simulink model "Ex7_4"  (Simulink 6.0)
settings: Solver=ode4  SolverMode=SingleTasking  StartTime=0.0  StopTime=200*Ts  RelTol=1e-3  AbsTol=1e-6
undefined symbols (not defined in the file or in its folder): Ampl, finrad, gainerror, offset, phasejitter, Ts
libraries: simulink x2
settings Model: Creator=francomaloberti  LastModifiedBy=Cri  ExtModeAutoUpdateStatusClock=off
settings DataIOCC: LimitDataPoints=off  SignalLoggingName=sigsOut
settings OptimizationCC: BooleanDataType=off  InlineInvariantSignals=off
settings DebuggingCC: SolverPrmCheckMsg=none
settings HardwareCC: TargetUnknown=on

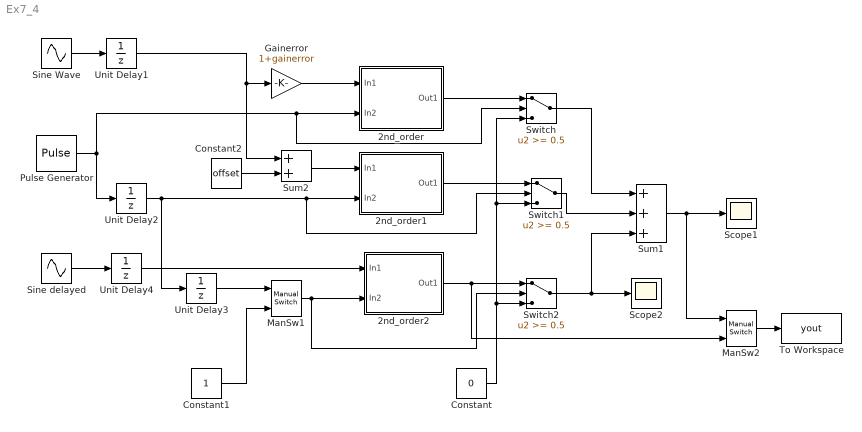
== system Ex7_4 ==
  2nd_order : Subsystem
      mask Display:
      | plot([20 10 20 10 20 30 40 20], [35 35 25 15 15 35 15 15])
      | port_label('input', 1, 'in');
      | port_label('input', 2, 'ck')
  2nd_order1 : Subsystem
      mask Display:
      | plot([20 10 20 10 20 30 40 20], [35 35 25 15 15 35 15 15])
      | port_label('input', 1, 'in');
      | port_label('input', 2, 'ck')
  2nd_order2 : Subsystem
      mask Display:
      | plot([20 10 20 10 20 30 40 20], [35 35 25 15 15 35 15 15])
      | port_label('input', 1, 'in');
      | port_label('input', 2, 'ck')
  Constant : Constant  Value=0
  Constant1 : Constant
  Constant2 : Constant  Value=offset
  Gainerror : Gain  Gain=1+gainerror
  ManSw1 : simulink/Signal Routing/Manual Switch  sw=1  action=0
  ManSw2 : simulink/Signal Routing/Manual Switch  sw=1  action=0
  Pulse Generator : DiscretePulseGenerator  PulseType=Time based  Period=3*Ts  PulseWidth=100/3
  Scope1 : Scope
      settings: TickLabels=on  DataFormat=Array
  Scope2 : Scope
      settings: TickLabels=on  SaveName=ScopeData2  DataFormat=Array
  Sine Wave : Sin  Amplitude=Ampl  Frequency=finrad  SampleTime=0
  Sine delayed : Sin  Amplitude=Ampl  Frequency=finrad  Phase=phasejitter  SampleTime=0
  Sum1 : Sum  Inputs=+++  SaturateOnIntegerOverflow=on  InputSameDT=on
  Sum2 : Sum  SaturateOnIntegerOverflow=on  InputSameDT=on
  Switch : Switch  Threshold=0.5
  Switch1 : Switch  Threshold=0.5
  Switch2 : Switch  Threshold=0.5
  To Workspace : ToWorkspace  VariableName=yout  SampleTime=-1  SaveFormat=Array
  Unit Delay{1..4} (4 alike) : UnitDelay  SampleTime=Ts
  wires:
  Sine Wave/1 -> Unit Delay1/1
  Pulse Generator/1 -> Unit Delay2/1, 2nd_order/2(In2), Switch/2
  Unit Delay1/1 -> Sum2/1, Gainerror/1
  Sum1/1 -> Scope1/1, ManSw2/1
  2nd_order/1(Out1) -> Switch/1
  2nd_order1/1(Out1) -> Switch1/1
  2nd_order2/1(Out1) -> ManSw2/2, Switch2/1
  Switch/1 -> Sum1/1
  Switch1/1 -> Sum1/2
  Constant/1 -> Switch2/3, Switch1/3, Switch/3
  Switch2/1 -> Scope2/1, Sum1/3
  Unit Delay2/1 -> Unit Delay3/1, Switch1/2, 2nd_order1/2(In2)
  ManSw1/1 -> Switch2/2, 2nd_order2/2(In2)
  Unit Delay3/1 -> ManSw1/1
  Constant1/1 -> ManSw1/2
  ManSw2/1 -> To Workspace/1
  Sum2/1 -> 2nd_order1/1(In1)
  Sine delayed/1 -> Unit Delay4/1
  Unit Delay4/1 -> 2nd_order2/1(In1)
  Constant2/1 -> Sum2/2
  Gainerror/1 -> 2nd_order/1(In1)

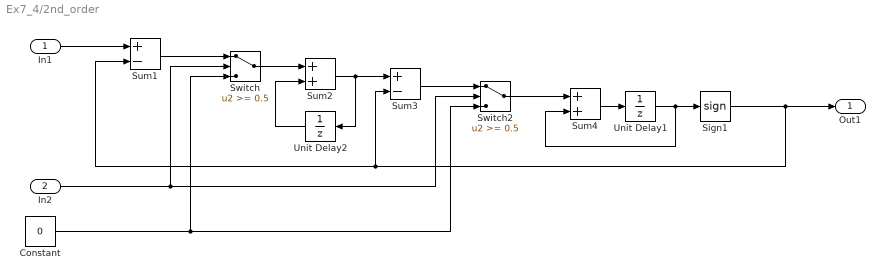
== system Ex7_4/2nd_order ==
  In1 : Inport  Port=1  LatchInput=off
  In2 : Inport  Port=2  LatchInput=off
  Constant : Constant  Value=0
  Sign1 : Signum
  Sum1 : Sum  Inputs=+-  SaturateOnIntegerOverflow=on  InputSameDT=on
  Sum2 : Sum  SaturateOnIntegerOverflow=on  InputSameDT=on
  Sum3 : Sum  Inputs=+-  SaturateOnIntegerOverflow=on  InputSameDT=on
  Sum4 : Sum  SaturateOnIntegerOverflow=on  InputSameDT=on
  Switch : Switch  Threshold=0.5
  Switch2 : Switch  Threshold=0.5
  Unit Delay1 : UnitDelay  SampleTime=Ts
  Unit Delay2 : UnitDelay  Orientation=left  SampleTime=Ts
  Out1 : Outport
  wires:
  Constant/1 -> Switch/3, Switch2/3
  In2/1 -> Switch/2, Switch2/2
  Sum2/1 -> Unit Delay2/1, Sum3/1
  Unit Delay2/1 -> Sum2/2
  Sum4/1 -> Unit Delay1/1
  Unit Delay1/1 -> Sum4/2, Sign1/1
  Switch2/1 -> Sum4/1
  Sum3/1 -> Switch2/1
  In1/1 -> Sum1/1
  Sum1/1 -> Switch/1
  Switch/1 -> Sum2/1
  Sign1/1 -> Sum1/2, Sum3/2, Out1/1

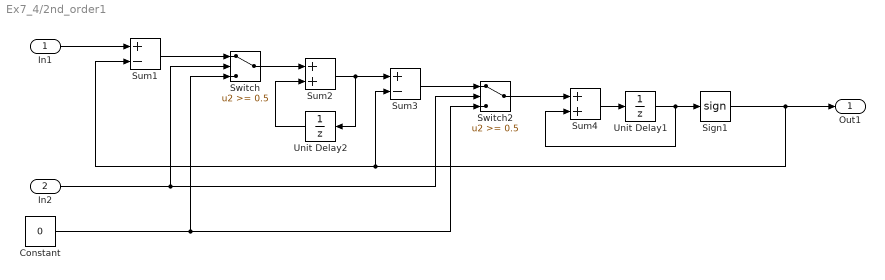
== system Ex7_4/2nd_order1 ==
  In1 : Inport  Port=1  LatchInput=off
  In2 : Inport  Port=2  LatchInput=off
  Constant : Constant  Value=0
  Sign1 : Signum
  Sum1 : Sum  Inputs=+-  SaturateOnIntegerOverflow=on  InputSameDT=on
  Sum2 : Sum  SaturateOnIntegerOverflow=on  InputSameDT=on
  Sum3 : Sum  Inputs=+-  SaturateOnIntegerOverflow=on  InputSameDT=on
  Sum4 : Sum  SaturateOnIntegerOverflow=on  InputSameDT=on
  Switch : Switch  Threshold=0.5
  Switch2 : Switch  Threshold=0.5
  Unit Delay1 : UnitDelay  SampleTime=Ts
  Unit Delay2 : UnitDelay  Orientation=left  SampleTime=Ts
  Out1 : Outport
  wires:
  Constant/1 -> Switch/3, Switch2/3
  In2/1 -> Switch/2, Switch2/2
  Sum2/1 -> Unit Delay2/1, Sum3/1
  Unit Delay2/1 -> Sum2/2
  Sum4/1 -> Unit Delay1/1
  Unit Delay1/1 -> Sum4/2, Sign1/1
  Switch2/1 -> Sum4/1
  Sum3/1 -> Switch2/1
  In1/1 -> Sum1/1
  Sum1/1 -> Switch/1
  Switch/1 -> Sum2/1
  Sign1/1 -> Sum1/2, Sum3/2, Out1/1

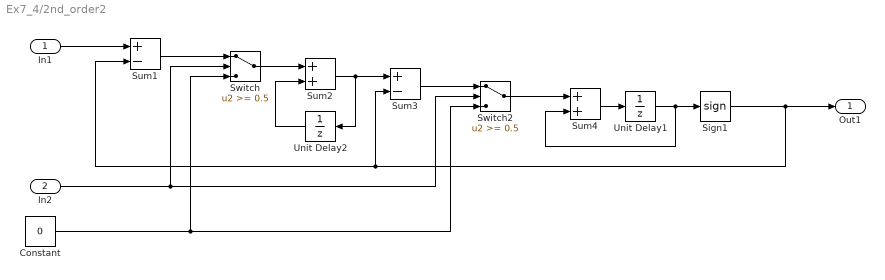
== system Ex7_4/2nd_order2 ==
  In1 : Inport  Port=1  LatchInput=off
  In2 : Inport  Port=2  LatchInput=off
  Constant : Constant  Value=0
  Sign1 : Signum
  Sum1 : Sum  Inputs=+-  SaturateOnIntegerOverflow=on  InputSameDT=on
  Sum2 : Sum  SaturateOnIntegerOverflow=on  InputSameDT=on
  Sum3 : Sum  Inputs=+-  SaturateOnIntegerOverflow=on  InputSameDT=on
  Sum4 : Sum  SaturateOnIntegerOverflow=on  InputSameDT=on
  Switch : Switch  Threshold=0.5
  Switch2 : Switch  Threshold=0.5
  Unit Delay1 : UnitDelay  SampleTime=Ts
  Unit Delay2 : UnitDelay  Orientation=left  SampleTime=Ts
  Out1 : Outport
  wires:
  Constant/1 -> Switch/3, Switch2/3
  In2/1 -> Switch/2, Switch2/2
  Sum2/1 -> Unit Delay2/1, Sum3/1
  Unit Delay2/1 -> Sum2/2
  Sum4/1 -> Unit Delay1/1
  Unit Delay1/1 -> Sum4/2, Sign1/1
  Switch2/1 -> Sum4/1
  Sum3/1 -> Switch2/1
  In1/1 -> Sum1/1
  Sum1/1 -> Switch/1
  Switch/1 -> Sum2/1
  Sign1/1 -> Sum1/2, Sum3/2, Out1/1
